simulink model "Driver_Model"  (R2016b)
settings: Solver=FixedStepDiscrete  StartTime=0.0  StopTime=inf  FixedStep=DrvrMdl.tiSimnTiStep_C.Value  RelTol=1e-3  EnableMultiTasking=on
settings Model: Creator=m01wolf  LastModifiedBy=bunver
settings DataIOCC: SaveFormat=StructureWithTime  SaveOutput=off  DSMLogging=off  VisualizeSimOutput=off  SaveTime=off  StateSaveName=Results  SignalLoggingName=Results
settings OptimizationCC: BlockReduction=off  ConditionallyExecuteInputs=off  LifeSpan=inf
settings DebuggingCC: AllowSymbolicDim=off  SFUnexpectedBacktrackingDiag=warning  SFNoUnconditionalDefaultTransitionDiag=warning  SFExecutionAtInitializationDiag=none
settings ModelReferenceCC: ModelReferenceNumInstancesAllowed=Single  PropagateSignalLabelsOutOfModel=off
settings GRTTargetCC: TargetLangStandard=C89/C90 (ANSI)
settings ConfigComp: CovMetricSettings=dw  CovHtmlReporting=on  CovSaveCumulativeToWorkspaceVar=on  CovSaveSingleToWorkspaceVar=on  CovExternalEMLEnable=off

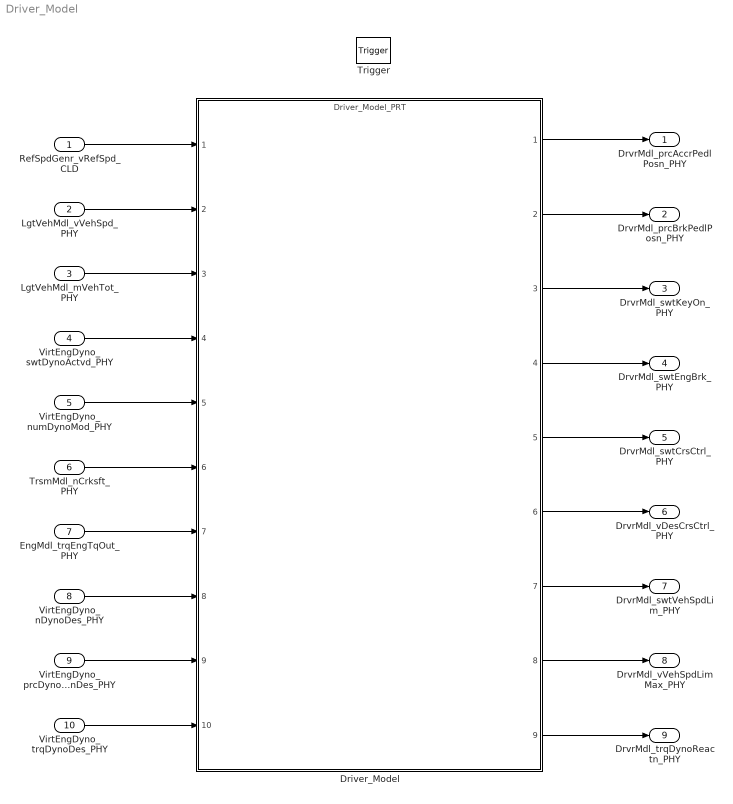
== system Driver_Model ==
  RefSpdGenr_vRefSpd_CLD : Inport
  LgtVehMdl_vVehSpd_PHY : Inport  Port=2
  LgtVehMdl_mVehTot_PHY : Inport  Port=3
  VirtEngDyno_swtDynoActvd_PHY : Inport  Port=4
  VirtEngDyno_numDynoMod_PHY : Inport  Port=5
  TrsmMdl_nCrksft_PHY : Inport  Port=6
  EngMdl_trqEngTqOut_PHY : Inport  Port=7
  VirtEngDyno_nDynoDes_PHY : Inport  Port=8
  VirtEngDyno_prcDynoAccrPedlPosnDes_PHY : Inport  Port=9
  VirtEngDyno_trqDynoDes_PHY : Inport  Port=10
  Trigger : TriggerPort  TriggerType=function-call  VariantControl=Variant  PortDimensions=1
  Driver_Model : ModelReference  ModelNameDialog=Driver_Model_PRT.slxp  ModelReferenceVersion=1.229  CopyOfModelProtected=on
  DrvrMdl_prcAccrPedlPosn_PHY : Outport
  DrvrMdl_prcBrkPedlPosn_PHY : Outport  Port=2
  DrvrMdl_swtKeyOn_PHY : Outport  Port=3
  DrvrMdl_swtEngBrk_PHY : Outport  Port=4
  DrvrMdl_swtCrsCtrl_PHY : Outport  Port=5
  DrvrMdl_vDesCrsCtrl_PHY : Outport  Port=6
  DrvrMdl_swtVehSpdLim_PHY : Outport  Port=7
  DrvrMdl_vVehSpdLimMax_PHY : Outport  Port=8
  DrvrMdl_trqDynoReactn_PHY : Outport  Port=9
  wires:
  RefSpdGenr_vRefSpd_CLD/1 -> Driver_Model/1
  LgtVehMdl_vVehSpd_PHY/1 -> Driver_Model/2
  LgtVehMdl_mVehTot_PHY/1 -> Driver_Model/3
  VirtEngDyno_swtDynoActvd_PHY/1 -> Driver_Model/4
  VirtEngDyno_trqDynoDes_PHY/1 -> Driver_Model/10
  VirtEngDyno_numDynoMod_PHY/1 -> Driver_Model/5
  TrsmMdl_nCrksft_PHY/1 -> Driver_Model/6
  EngMdl_trqEngTqOut_PHY/1 -> Driver_Model/7
  VirtEngDyno_nDynoDes_PHY/1 -> Driver_Model/8
  VirtEngDyno_prcDynoAccrPedlPosnDes_PHY/1 -> Driver_Model/9
  Driver_Model/9 -> DrvrMdl_trqDynoReactn_PHY/1
  Driver_Model/1 -> DrvrMdl_prcAccrPedlPosn_PHY/1
  Driver_Model/7 -> DrvrMdl_swtVehSpdLim_PHY/1
  Driver_Model/3 -> DrvrMdl_swtKeyOn_PHY/1
  Driver_Model/4 -> DrvrMdl_swtEngBrk_PHY/1
  Driver_Model/2 -> DrvrMdl_prcBrkPedlPosn_PHY/1
  Driver_Model/8 -> DrvrMdl_vVehSpdLimMax_PHY/1
  Driver_Model/6 -> DrvrMdl_vDesCrsCtrl_PHY/1
  Driver_Model/5 -> DrvrMdl_swtCrsCtrl_PHY/1
